simulink model "bump'em_control_system"  (R2018a)
settings: Solver=ode4  StartTime=0.0  StopTime=Inf  FixedStep=0.001  RelTol=1e-3
PostLoadFcn:
  | , if any(exist('dsrtsu_mdlpostloadfcn', 'file') == [2, 3, 6]), try dsrtsu_mdlpostloadfcn('Execute', bdroot); catch fprintf('Error in PostLoadFcn (dsrtsu_mdlpostloadfcn) for model "%s":\n %s\n', bdroot, lasterr); end, end,
libraries: rti1202lib_dac_class1 x4, simulink x4, dsparch4 x2, rti1202lib_adc_class1 x2
(part 2 of 2)

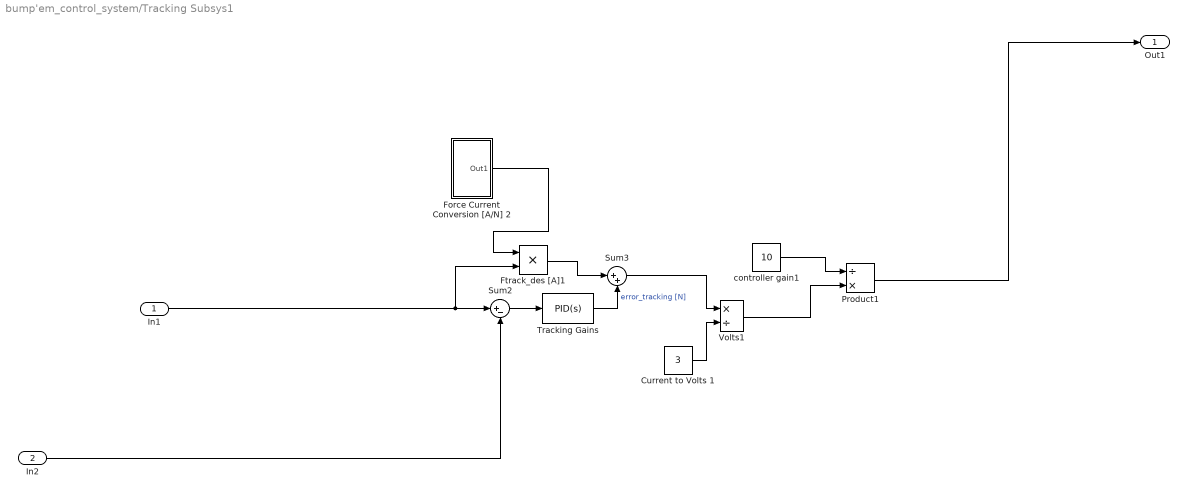
== system bump'em_control_system/Tracking Subsys1 ==
  In1 : Inport
  In2 : Inport  Port=2
  Current to Volts 1 : Constant  Value=3
  Force Current Conversion [A/N] 2 : Subsystem
  Ftrack_des [A]1 : Product
  Product1 : Product  Inputs=/*
  Sum2 : Sum  Inputs=|+-
  Sum3 : Sum  Inputs=|++
  Tracking Gains : simulink/Continuous/PID Controller  Controller=PID  TimeDomain=Continuous-time  SampleTime=-1  IntegratorMethod=Forward Euler  FilterMethod=Forward Euler  Form=Parallel  UseFilter=on  ControllerParametersSource=internal  P=0  I=0  D=0  N=100  InitialConditionSource=internal  InitialConditionForIntegrator=0  InitialConditionForFilter=0  ExternalReset=none  LimitOutput=off  UpperSaturationLimit=inf  LowerSaturationLimit=-inf  LinearizeAsGain=on  AntiWindupMode=none  Kb=1  TrackingMode=off  Kt=1  PParamMin=[]  PParamMax=[]  IParamMin=[]  IParamMax=[]  DParamMin=[]  DParamMax=[]  NParamMin=[]  NParamMax=[]  KbParamMin=[]  KbParamMax=[]  KtParamMin=[]  KtParamMax=[]  POutMin=[]  POutMax=[]  IOutMin=[]  IOutMax=[]  DOutMin=[]  DOutMax=[]  NOutMin=[]  NOutMax=[]  KbOutMin=[]  KbOutMax=[]  KtOutMin=[]  KtOutMax=[]  IntegratorOutMin=[]  IntegratorOutMax=[]  FilterOutMin=[]  FilterOutMax=[]  SumOutMin=[]  SumOutMax=[]  SumI1OutMin=[]  SumI1OutMax=[]  SumI2OutMin=[]  SumI2OutMax=[]  SumI3OutMin=[]  SumI3OutMax=[]  SumDOutMin=[]  SumDOutMax=[]  SaturationOutMin=[]  SaturationOutMax=[]  IntegratorContinuousStateAttributes=''  IntegratorStateMustResolveToSignalObject=off  IntegratorRTWStateStorageClass=Auto  FilterContinuousStateAttributes=''  FilterStateMustResolveToSignalObject=off  FilterRTWStateStorageClass=Auto  DifferentiatorICPrevScaledInput=0  DifferentiatorOutMin=[]  DifferentiatorOutMax=[]  FilterDiffOutCoefMin=[]  FilterDiffOutCoefMax=[]  SumDenOutMin=[]  SumDenOutMax=[]  SumNumOutMin=[]  SumNumOutMax=[]  ReciprocalOutMin=[]  ReciprocalOutMax=[]  DivideOutMin=[]  DivideOutMax=[]  TunerSelectOption=Transfer Function Based (PID Tuner App)
  Volts1 : Product  Inputs=*/
  controller gain1 : Constant  Value=10
  Out1 : Outport  VectorParamsAs1DForOutWhenUnconnected=on
  wires:
  controller gain1/1 -> Product1/1
  Tracking Gains/1 -> Sum3/2  "error_tracking [N]"
  Current to Volts 1/1 -> Volts1/2
  In1/1 -> Ftrack_des [A]1/2, Sum2/1
  Volts1/1 -> Product1/2
  Sum3/1 -> Volts1/1
  Sum2/1 -> Tracking Gains/1
  Product1/1 -> Out1/1
  In2/1 -> Sum2/2
  Ftrack_des [A]1/1 -> Sum3/1
  Force Current Conversion [A/N] 2/1(Out1) -> Ftrack_des [A]1/1

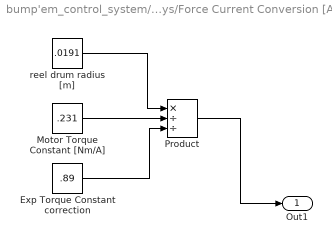
== system bump'em_control_system/Pertubration Subsys/Force Current Conversion [A//N] 1 ==
  Exp Torque Constant correction : Constant  Value=.89
  "Motor Torque Constant [Nm/A] " : Constant  Value=.231
  Product : Product  Inputs=*//
  "reel drum radius [m] " : Constant  Value=.0191
  Out1 : Outport
  wires:
  "Motor Torque Constant [Nm/A] "/1 -> Product/2
  Product/1 -> Out1/1
  "reel drum radius [m] "/1 -> Product/1
  Exp Torque Constant correction/1 -> Product/3

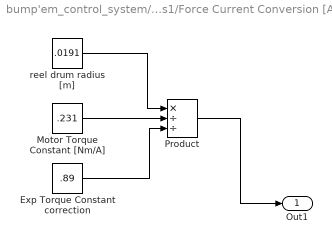
== system bump'em_control_system/Pertubration Subsys1/Force Current Conversion [A//N] 1 ==
  Exp Torque Constant correction : Constant  Value=.89
  "Motor Torque Constant [Nm/A] " : Constant  Value=.231
  Product : Product  Inputs=*//
  "reel drum radius [m] " : Constant  Value=.0191
  Out1 : Outport
  wires:
  "Motor Torque Constant [Nm/A] "/1 -> Product/2
  Product/1 -> Out1/1
  "reel drum radius [m] "/1 -> Product/1
  Exp Torque Constant correction/1 -> Product/3

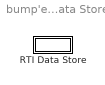
== system bump'em_control_system/RTI Data/RTI Data Store ==
  RTI Data Store : Subsystem  mask(RTI_DATA_STORE){}
      mask help:
      | RTI Data Store Block. This block is used by RTI to store internal model dependent data. Deleting this block will result in data loss.
      |
      | NEVER DELETE, COPY, OR MODIFY THIS BLOCK!
      mask Help:
      | RTI Data Store Block. This block is used by RTI to store internal model dependent data. Deleting this block will result in data loss.
      | 
      | NEVER DELETE, COPY, OR MODIFY THIS BLOCK!
      mask Display: text(0.5, 0.5, ' ', 'HorizontalAlignment', 'center');

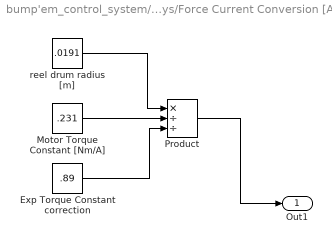
== system bump'em_control_system/Tracking Subsys/Force Current Conversion [A//N] 2 ==
  Exp Torque Constant correction : Constant  Value=.89
  "Motor Torque Constant [Nm/A] " : Constant  Value=.231
  Product : Product  Inputs=*//
  "reel drum radius [m] " : Constant  Value=.0191
  Out1 : Outport
  wires:
  "Motor Torque Constant [Nm/A] "/1 -> Product/2
  Product/1 -> Out1/1
  "reel drum radius [m] "/1 -> Product/1
  Exp Torque Constant correction/1 -> Product/3

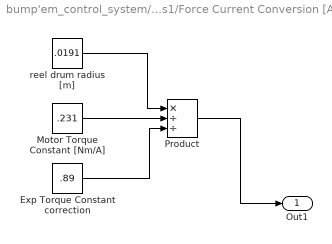
== system bump'em_control_system/Tracking Subsys1/Force Current Conversion [A//N] 2 ==
  Exp Torque Constant correction : Constant  Value=.89
  "Motor Torque Constant [Nm/A] " : Constant  Value=.231
  Product : Product  Inputs=*//
  "reel drum radius [m] " : Constant  Value=.0191
  Out1 : Outport
  wires:
  "Motor Torque Constant [Nm/A] "/1 -> Product/2
  Product/1 -> Out1/1
  "reel drum radius [m] "/1 -> Product/1
  Exp Torque Constant correction/1 -> Product/3

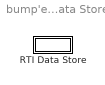
== system bump'em_control_system/RTI Data/RTI Data Store/RTI Data Store ==
  RTI Data Store : Subsystem  mask(RTI_DATA_STORE){}
      mask help:
      | RTI Data Store Block. This block is used by RTI to store internal model dependent data. Deleting this block will result in data loss.
      |
      | NEVER DELETE, COPY, OR MODIFY THIS BLOCK!
      mask Help:
      | RTI Data Store Block. This block is used by RTI to store internal model dependent data. Deleting this block will result in data loss.
      | 
      | NEVER DELETE, COPY, OR MODIFY THIS BLOCK!
      mask Display: text(0.5, 0.5, ' ', 'HorizontalAlignment', 'center');

== system bump'em_control_system/RTI Data/RTI Data Store/RTI Data Store/RTI Data Store ==
  RTI Data Store : Subsystem  mask(RTI_DATA_STORE){}
      mask help:
      | RTI Data Store Block. This block is used by RTI to store internal model dependent data. Deleting this block will result in data loss.
      |
      | NEVER DELETE, COPY, OR MODIFY THIS BLOCK!
      mask Help:
      | RTI Data Store Block. This block is used by RTI to store internal model dependent data. Deleting this block will result in data loss.
      | 
      | NEVER DELETE, COPY, OR MODIFY THIS BLOCK!
      mask Display: text(0.5, 0.5, ' ', 'HorizontalAlignment', 'center');

== system bump'em_control_system/RTI Data/RTI Data Store/RTI Data Store/RTI Data Store/RTI Data Store ==
